simulink model "SIT_RWSW"  (Simulink 8.8)
settings: Solver=VariableStepAuto  StartTime=0.0  StopTime=sim_par.t_end  RelTol=1e-3
libraries: POSTPROC x3, RWSW x1
settings Model: Creator=alger  LastModifiedBy=alger  SimulationMode=rapid-accelerator
settings DataIOCC: LimitDataPoints=off  SaveFormat=Dataset  SignalLoggingSaveFormat=Dataset
settings OptimizationCC: LifeSpan=auto
settings DebuggingCC: UnderspecifiedInitializationDetection=Simplified  MergeDetectMultiDrivingBlocksExec=error  FcnCallInpInsideContextMsg=error  StateNameClashWarn=none  SFUnexpectedBacktrackingDiag=error  SFNoUnconditionalDefaultTransitionDiag=error  SFExecutionAtInitializationDiag=warning
settings HardwareCC: ProdBitPerPointer=64  ProdBitPerSizeT=64  ProdBitPerPtrDiffT=64  ProdLargestAtomicFloat=Float  ProdIntDivRoundTo=Zero  ProdEndianess=LittleEndian  ProdWordSize=64  ProdHWDeviceType=Intel->x86-64 (Windows64)
settings ModelReferenceCC: PropagateSignalLabelsOutOfModel=on
settings GRTTargetCC: TargetLangStandard=C99 (ISO)  GeneratePreprocessorConditionals=Use local settings  CombineOutputUpdateFcns=on  GRTInterface=off
settings ConfigComp: CovMetricSettings=dwe  CovHtmlReporting=off  CovSaveCumulativeToWorkspaceVar=off  CovSaveSingleToWorkspaceVar=off  CovExternalEMLEnable=on

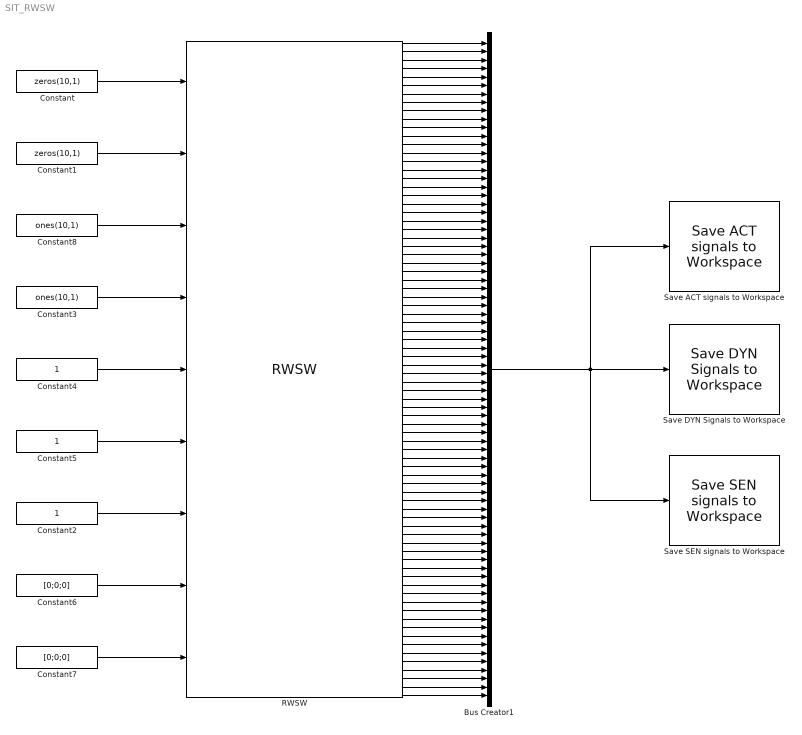
== system SIT_RWSW ==
  Bus Creator1 : BusCreator  Inputs=78
  Constant : Constant  Value=zeros(10,1)
  Constant1 : Constant  Value=zeros(10,1)
  Constant2 : Constant
  Constant3 : Constant  Value=ones(10,1)
  Constant4 : Constant
  Constant5 : Constant
  Constant6 : Constant  Value=[0;0;0]
  Constant7 : Constant  Value=[0;0;0]
  Constant8 : Constant  Value=ones(10,1)
  RWSW : RWSW/RWSW
  Save ACT signals to Workspace : POSTPROC/Save ACT signals to Workspace
  Save DYN Signals to Workspace : POSTPROC/Save DYN Signals to Workspace
  Save SEN signals to Workspace : POSTPROC/Save SEN signals to Workspace
  wires:
  Constant/1 -> RWSW/1
  Constant1/1 -> RWSW/2
  Constant3/1 -> RWSW/4
  Constant4/1 -> RWSW/5
  Constant5/1 -> RWSW/6
  Bus Creator1/1 -> Save SEN signals to Workspace/1, Save DYN Signals to Workspace/1, Save ACT signals to Workspace/1
  RWSW/14 -> Bus Creator1/14
  RWSW/39 -> Bus Creator1/39
  RWSW/41 -> Bus Creator1/41
  RWSW/42 -> Bus Creator1/42
  RWSW/44 -> Bus Creator1/44
  RWSW/46 -> Bus Creator1/46
  RWSW/5 -> Bus Creator1/5
  RWSW/1 -> Bus Creator1/1
  RWSW/23 -> Bus Creator1/23
  RWSW/25 -> Bus Creator1/25
  RWSW/30 -> Bus Creator1/30
  RWSW/33 -> Bus Creator1/33
  RWSW/36 -> Bus Creator1/36
  RWSW/12 -> Bus Creator1/12
  RWSW/17 -> Bus Creator1/17
  RWSW/20 -> Bus Creator1/20
  RWSW/28 -> Bus Creator1/28
  RWSW/11 -> Bus Creator1/11
  RWSW/9 -> Bus Creator1/9
  RWSW/16 -> Bus Creator1/16
  RWSW/31 -> Bus Creator1/31
  RWSW/47 -> Bus Creator1/47
  RWSW/10 -> Bus Creator1/10
  RWSW/32 -> Bus Creator1/32
  RWSW/3 -> Bus Creator1/3
  RWSW/27 -> Bus Creator1/27
  RWSW/37 -> Bus Creator1/37
  RWSW/22 -> Bus Creator1/22
  RWSW/29 -> Bus Creator1/29
  RWSW/7 -> Bus Creator1/7
  RWSW/8 -> Bus Creator1/8
  RWSW/15 -> Bus Creator1/15
  RWSW/21 -> Bus Creator1/21
  RWSW/34 -> Bus Creator1/34
  RWSW/35 -> Bus Creator1/35
  RWSW/2 -> Bus Creator1/2
  RWSW/18 -> Bus Creator1/18
  RWSW/19 -> Bus Creator1/19
  RWSW/26 -> Bus Creator1/26
  RWSW/40 -> Bus Creator1/40
  RWSW/43 -> Bus Creator1/43
  RWSW/13 -> Bus Creator1/13
  RWSW/45 -> Bus Creator1/45
  RWSW/24 -> Bus Creator1/24
  RWSW/4 -> Bus Creator1/4
  RWSW/6 -> Bus Creator1/6
  RWSW/38 -> Bus Creator1/38
  RWSW/61 -> Bus Creator1/61
  RWSW/53 -> Bus Creator1/53
  RWSW/49 -> Bus Creator1/49
  RWSW/70 -> Bus Creator1/70
  RWSW/72 -> Bus Creator1/72
  RWSW/55 -> Bus Creator1/55
  RWSW/64 -> Bus Creator1/64
  RWSW/68 -> Bus Creator1/68
  RWSW/56 -> Bus Creator1/56
  RWSW/48 -> Bus Creator1/48
  RWSW/59 -> Bus Creator1/59
  RWSW/51 -> Bus Creator1/51
  RWSW/60 -> Bus Creator1/60
  RWSW/67 -> Bus Creator1/67
  RWSW/71 -> Bus Creator1/71
  RWSW/52 -> Bus Creator1/52
  RWSW/73 -> Bus Creator1/73
  RWSW/54 -> Bus Creator1/54
  RWSW/62 -> Bus Creator1/62
  RWSW/50 -> Bus Creator1/50
  RWSW/66 -> Bus Creator1/66
  RWSW/69 -> Bus Creator1/69
  RWSW/57 -> Bus Creator1/57
  RWSW/65 -> Bus Creator1/65
  RWSW/58 -> Bus Creator1/58
  RWSW/63 -> Bus Creator1/63
  Constant8/1 -> RWSW/3
  Constant2/1 -> RWSW/7
  Constant6/1 -> RWSW/8
  Constant7/1 -> RWSW/9
  RWSW/77 -> Bus Creator1/77
  RWSW/76 -> Bus Creator1/76
  RWSW/74 -> Bus Creator1/74
  RWSW/75 -> Bus Creator1/75
  RWSW/78 -> Bus Creator1/78
